simulink model "W06_city_highway_cs"  (R2019a)
settings: Solver=ode5  StartTime=0.0  StopTime=inf  FixedStep=1/60  RelTol=1e-3
PreLoadFcn:
  | mbxruntime.callbacks.PreLoadFcn(bdroot);
PostLoadFcn:
  | mbxruntime.callbacks.PostLoadFcn(bdroot);
InitFcn:
  | mbxruntime.callbacks.InitFcn(bdroot);
StartFcn:
  | mbxruntime.callbacks.StartFcn(bdroot);
StopFcn:
  | mbxruntime.callbacks.StopFcn(bdroot);
model workspace: external: MAT-File .\W06_city_highway_cs_hws.mat (data not in the file)
undefined symbols (not defined in the file or in its folder): DiscIntNeverNeededParam, FovAzimuth, FovAzimuthDefined, FovElevation, FovElevationDefined, Header, InitImageOutputDir, LocationX, LocationXDefined, LocationY, LocationYDefined, LocationZ, LocationZDefined, Orientation, OrientationPitch, OrientationPitchDefined, OrientationRoll, OrientationRollDefined, OrientationYaw, OrientationYawDefined, Poses, Poses_SL_Info, Position, W06_city_highway_cs_0270c22595f3b0e3, W06_city_highway_cs_086892688dd32ddc, W06_city_highway_cs_328c49ac39fca66b, W06_city_highway_cs_35ce05381b8ebe8c, W06_city_highway_cs_47b384f162638175, W06_city_highway_cs_766f76ce4de94dd5, W06_city_highway_cs_8c547f67cb81ffba, W06_city_highway_cs_aed52f2a7724a4f9, W06_city_highway_cs_Audi_A8_Sedan_1_Path_pathUniqueID, W06_city_highway_cs_b74cbb1f9f7331b5, W06_city_highway_cs_Citroen_C3_Hatchback_1_Path_pathUniqueID, W06_city_highway_cs_d395f8835e0c28b3, W06_city_highway_cs_e5f9d1759e19e2b4, W06_city_highway_cs_Toyota_Previa_MPV_1_Path_pathUniqueID
libraries: adeye_lib x26, simulink_extras x24, robotlib x7, sharedtransform x4, PreScanSimulinkLibrary x2, PreScanUsefulBlocks x1
(part 8 of 8)

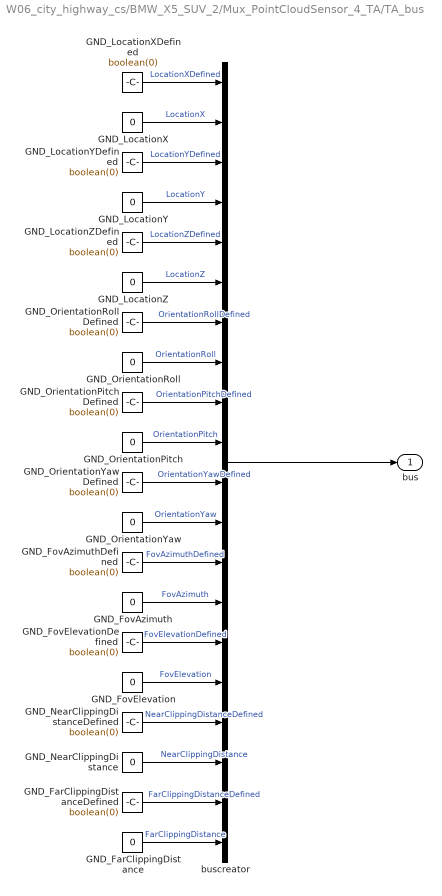
== system W06_city_highway_cs/BMW_X5_SUV_2/Mux_PointCloudSensor_4_TA/TA_bus ==
  GND_FarClippingDistance : Constant  Value=0
  GND_FarClippingDistanceDefined : Constant  Value=boolean(0)
  GND_FovAzimuth : Constant  Value=0
  GND_FovAzimuthDefined : Constant  Value=boolean(0)
  GND_FovElevation : Constant  Value=0
  GND_FovElevationDefined : Constant  Value=boolean(0)
  GND_LocationX : Constant  Value=0
  GND_LocationXDefined : Constant  Value=boolean(0)
  GND_LocationY : Constant  Value=0
  GND_LocationYDefined : Constant  Value=boolean(0)
  GND_LocationZ : Constant  Value=0
  GND_LocationZDefined : Constant  Value=boolean(0)
  GND_NearClippingDistance : Constant  Value=0
  GND_NearClippingDistanceDefined : Constant  Value=boolean(0)
  GND_OrientationPitch : Constant  Value=0
  GND_OrientationPitchDefined : Constant  Value=boolean(0)
  GND_OrientationRoll : Constant  Value=0
  GND_OrientationRollDefined : Constant  Value=boolean(0)
  GND_OrientationYaw : Constant  Value=0
  GND_OrientationYawDefined : Constant  Value=boolean(0)
  buscreator : BusCreator  Inputs=20  OutDataTypeStr=Bus: PRESCAN_PCS_TA_DATA  NonVirtualBus=on
  bus : Outport  OutDataTypeStr=Bus: PRESCAN_PCS_TA_DATA
  wires:
  GND_LocationXDefined/1 -> buscreator/1  "LocationXDefined"
  GND_LocationX/1 -> buscreator/2  "LocationX"
  GND_LocationYDefined/1 -> buscreator/3  "LocationYDefined"
  GND_LocationY/1 -> buscreator/4  "LocationY"
  GND_LocationZDefined/1 -> buscreator/5  "LocationZDefined"
  GND_LocationZ/1 -> buscreator/6  "LocationZ"
  GND_OrientationRollDefined/1 -> buscreator/7  "OrientationRollDefined"
  GND_OrientationRoll/1 -> buscreator/8  "OrientationRoll"
  GND_OrientationPitchDefined/1 -> buscreator/9  "OrientationPitchDefined"
  GND_OrientationPitch/1 -> buscreator/10  "OrientationPitch"
  GND_OrientationYawDefined/1 -> buscreator/11  "OrientationYawDefined"
  GND_OrientationYaw/1 -> buscreator/12  "OrientationYaw"
  GND_FovAzimuthDefined/1 -> buscreator/13  "FovAzimuthDefined"
  GND_FovAzimuth/1 -> buscreator/14  "FovAzimuth"
  GND_FovElevationDefined/1 -> buscreator/15  "FovElevationDefined"
  GND_FovElevation/1 -> buscreator/16  "FovElevation"
  GND_NearClippingDistanceDefined/1 -> buscreator/17  "NearClippingDistanceDefined"
  GND_NearClippingDistance/1 -> buscreator/18  "NearClippingDistance"
  GND_FarClippingDistanceDefined/1 -> buscreator/19  "FarClippingDistanceDefined"
  GND_FarClippingDistance/1 -> buscreator/20  "FarClippingDistance"
  buscreator/1 -> bus/1

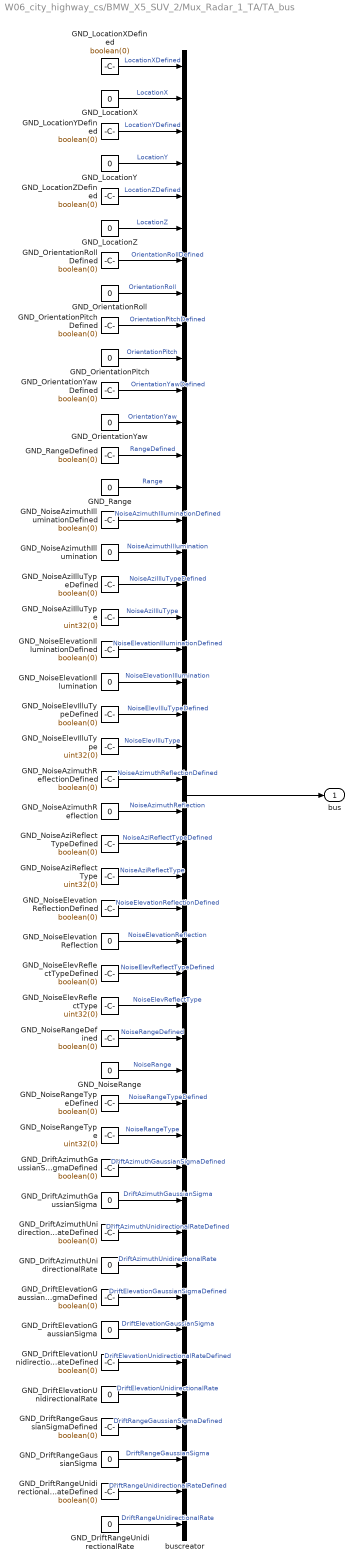
== system W06_city_highway_cs/BMW_X5_SUV_2/Mux_Radar_1_TA/TA_bus ==
  GND_DriftAzimuthGaussianSigma : Constant  Value=0
  GND_DriftAzimuthGaussianSigmaDefined : Constant  Value=boolean(0)
  GND_DriftAzimuthUnidirectionalRate : Constant  Value=0
  GND_DriftAzimuthUnidirectionalRateDefined : Constant  Value=boolean(0)
  GND_DriftElevationGaussianSigma : Constant  Value=0
  GND_DriftElevationGaussianSigmaDefined : Constant  Value=boolean(0)
  GND_DriftElevationUnidirectionalRate : Constant  Value=0
  GND_DriftElevationUnidirectionalRateDefined : Constant  Value=boolean(0)
  GND_DriftRangeGaussianSigma : Constant  Value=0
  GND_DriftRangeGaussianSigmaDefined : Constant  Value=boolean(0)
  GND_DriftRangeUnidirectionalRate : Constant  Value=0
  GND_DriftRangeUnidirectionalRateDefined : Constant  Value=boolean(0)
  GND_LocationX : Constant  Value=0
  GND_LocationXDefined : Constant  Value=boolean(0)
  GND_LocationY : Constant  Value=0
  GND_LocationYDefined : Constant  Value=boolean(0)
  GND_LocationZ : Constant  Value=0
  GND_LocationZDefined : Constant  Value=boolean(0)
  GND_NoiseAziIlluType : Constant  Value=uint32(0)
  GND_NoiseAziIlluTypeDefined : Constant  Value=boolean(0)
  GND_NoiseAziReflectType : Constant  Value=uint32(0)
  GND_NoiseAziReflectTypeDefined : Constant  Value=boolean(0)
  GND_NoiseAzimuthIllumination : Constant  Value=0
  GND_NoiseAzimuthIlluminationDefined : Constant  Value=boolean(0)
  GND_NoiseAzimuthReflection : Constant  Value=0
  GND_NoiseAzimuthReflectionDefined : Constant  Value=boolean(0)
  GND_NoiseElevIlluType : Constant  Value=uint32(0)
  GND_NoiseElevIlluTypeDefined : Constant  Value=boolean(0)
  GND_NoiseElevReflectType : Constant  Value=uint32(0)
  GND_NoiseElevReflectTypeDefined : Constant  Value=boolean(0)
  GND_NoiseElevationIllumination : Constant  Value=0
  GND_NoiseElevationIlluminationDefined : Constant  Value=boolean(0)
  GND_NoiseElevationReflection : Constant  Value=0
  GND_NoiseElevationReflectionDefined : Constant  Value=boolean(0)
  GND_NoiseRange : Constant  Value=0
  GND_NoiseRangeDefined : Constant  Value=boolean(0)
  GND_NoiseRangeType : Constant  Value=uint32(0)
  GND_NoiseRangeTypeDefined : Constant  Value=boolean(0)
  GND_OrientationPitch : Constant  Value=0
  GND_OrientationPitchDefined : Constant  Value=boolean(0)
  GND_OrientationRoll : Constant  Value=0
  GND_OrientationRollDefined : Constant  Value=boolean(0)
  GND_OrientationYaw : Constant  Value=0
  GND_OrientationYawDefined : Constant  Value=boolean(0)
  GND_Range : Constant  Value=0
  GND_RangeDefined : Constant  Value=boolean(0)
  buscreator : BusCreator  Inputs=46  OutDataTypeStr=Bus: PRESCAN_SCANNERSENSOR_TA  NonVirtualBus=on
  bus : Outport  OutDataTypeStr=Bus: PRESCAN_SCANNERSENSOR_TA
  wires:
  GND_LocationXDefined/1 -> buscreator/1  "LocationXDefined"
  GND_LocationX/1 -> buscreator/2  "LocationX"
  GND_LocationYDefined/1 -> buscreator/3  "LocationYDefined"
  GND_LocationY/1 -> buscreator/4  "LocationY"
  GND_LocationZDefined/1 -> buscreator/5  "LocationZDefined"
  GND_LocationZ/1 -> buscreator/6  "LocationZ"
  GND_OrientationRollDefined/1 -> buscreator/7  "OrientationRollDefined"
  GND_OrientationRoll/1 -> buscreator/8  "OrientationRoll"
  GND_OrientationPitchDefined/1 -> buscreator/9  "OrientationPitchDefined"
  GND_OrientationPitch/1 -> buscreator/10  "OrientationPitch"
  GND_OrientationYawDefined/1 -> buscreator/11  "OrientationYawDefined"
  GND_OrientationYaw/1 -> buscreator/12  "OrientationYaw"
  GND_RangeDefined/1 -> buscreator/13  "RangeDefined"
  GND_Range/1 -> buscreator/14  "Range"
  GND_NoiseAzimuthIlluminationDefined/1 -> buscreator/15  "NoiseAzimuthIlluminationDefined"
  GND_NoiseAzimuthIllumination/1 -> buscreator/16  "NoiseAzimuthIllumination"
  GND_NoiseAziIlluTypeDefined/1 -> buscreator/17  "NoiseAziIlluTypeDefined"
  GND_NoiseAziIlluType/1 -> buscreator/18  "NoiseAziIlluType"
  GND_NoiseElevationIlluminationDefined/1 -> buscreator/19  "NoiseElevationIlluminationDefined"
  GND_NoiseElevationIllumination/1 -> buscreator/20  "NoiseElevationIllumination"
  GND_NoiseElevIlluTypeDefined/1 -> buscreator/21  "NoiseElevIlluTypeDefined"
  GND_NoiseElevIlluType/1 -> buscreator/22  "NoiseElevIlluType"
  GND_NoiseAzimuthReflectionDefined/1 -> buscreator/23  "NoiseAzimuthReflectionDefined"
  GND_NoiseAzimuthReflection/1 -> buscreator/24  "NoiseAzimuthReflection"
  GND_NoiseAziReflectTypeDefined/1 -> buscreator/25  "NoiseAziReflectTypeDefined"
  GND_NoiseAziReflectType/1 -> buscreator/26  "NoiseAziReflectType"
  GND_NoiseElevationReflectionDefined/1 -> buscreator/27  "NoiseElevationReflectionDefined"
  GND_NoiseElevationReflection/1 -> buscreator/28  "NoiseElevationReflection"
  GND_NoiseElevReflectTypeDefined/1 -> buscreator/29  "NoiseElevReflectTypeDefined"
  GND_NoiseElevReflectType/1 -> buscreator/30  "NoiseElevReflectType"
  GND_NoiseRangeDefined/1 -> buscreator/31  "NoiseRangeDefined"
  GND_NoiseRange/1 -> buscreator/32  "NoiseRange"
  GND_NoiseRangeTypeDefined/1 -> buscreator/33  "NoiseRangeTypeDefined"
  GND_NoiseRangeType/1 -> buscreator/34  "NoiseRangeType"
  GND_DriftAzimuthGaussianSigmaDefined/1 -> buscreator/35  "DriftAzimuthGaussianSigmaDefined"
  GND_DriftAzimuthGaussianSigma/1 -> buscreator/36  "DriftAzimuthGaussianSigma"
  GND_DriftAzimuthUnidirectionalRateDefined/1 -> buscreator/37  "DriftAzimuthUnidirectionalRateDefined"
  GND_DriftAzimuthUnidirectionalRate/1 -> buscreator/38  "DriftAzimuthUnidirectionalRate"
  GND_DriftElevationGaussianSigmaDefined/1 -> buscreator/39  "DriftElevationGaussianSigmaDefined"
  GND_DriftElevationGaussianSigma/1 -> buscreator/40  "DriftElevationGaussianSigma"
  GND_DriftElevationUnidirectionalRateDefined/1 -> buscreator/41  "DriftElevationUnidirectionalRateDefined"
  GND_DriftElevationUnidirectionalRate/1 -> buscreator/42  "DriftElevationUnidirectionalRate"
  GND_DriftRangeGaussianSigmaDefined/1 -> buscreator/43  "DriftRangeGaussianSigmaDefined"
  GND_DriftRangeGaussianSigma/1 -> buscreator/44  "DriftRangeGaussianSigma"
  GND_DriftRangeUnidirectionalRateDefined/1 -> buscreator/45  "DriftRangeUnidirectionalRateDefined"
  GND_DriftRangeUnidirectionalRate/1 -> buscreator/46  "DriftRangeUnidirectionalRate"
  buscreator/1 -> bus/1

== system W06_city_highway_cs/BMW_X5_SUV_2/SELF_Demux/compas converter ==
  rotz [rad] : Inport
  cart2compas : Subsystem
  rad2deg : Gain  Gain=180/pi
  heading [deg] : Outport
  wires:
  rad2deg/1 -> cart2compas/1(Angle [deg])
  rotz [rad]/1 -> rad2deg/1
  cart2compas/1(heading [deg]) -> heading [deg]/1

== system W06_city_highway_cs/Citroen_C3_Hatchback_1/SELF_Demux/compas converter ==
  rotz [rad] : Inport
  cart2compas : Subsystem
  rad2deg : Gain  Gain=180/pi
  heading [deg] : Outport
  wires:
  rad2deg/1 -> cart2compas/1(Angle [deg])
  rotz [rad]/1 -> rad2deg/1
  cart2compas/1(heading [deg]) -> heading [deg]/1

== system W06_city_highway_cs/MercedesBenz_Actros_2541_L_6x2_1/SELF_Demux/compas converter ==
  rotz [rad] : Inport
  cart2compas : Subsystem
  rad2deg : Gain  Gain=180/pi
  heading [deg] : Outport
  wires:
  rad2deg/1 -> cart2compas/1(Angle [deg])
  rotz [rad]/1 -> rad2deg/1
  cart2compas/1(heading [deg]) -> heading [deg]/1

== system W06_city_highway_cs/Toyota_Previa_MPV_1/SELF_Demux/compas converter ==
  rotz [rad] : Inport
  cart2compas : Subsystem
  rad2deg : Gain  Gain=180/pi
  heading [deg] : Outport
  wires:
  rad2deg/1 -> cart2compas/1(Angle [deg])
  rotz [rad]/1 -> rad2deg/1
  cart2compas/1(heading [deg]) -> heading [deg]/1

== system W06_city_highway_cs/Audi_A8_Sedan_1/SELF_Demux/compas converter/cart2compas ==
  Angle [deg] : Inport
  Constant : Constant  Value=90
  Constant1 : Constant  Value=360
  Gain : Gain  Gain=1/360
  Gain1 : Gain  Gain=360
  Gain2 : Gain  Gain=-1
  Rounding Function : Rounding
  Sum : Sum  Inputs=|-+
  Sum1 : Sum  Inputs=-+|
  Sum2 : Sum  Inputs=++|
  heading [deg] : Outport
  wires:
  Gain/1 -> Rounding Function/1
  Rounding Function/1 -> Gain1/1
  Gain1/1 -> Sum/1
  Angle [deg]/1 -> Sum1/2
  Sum/1 -> Gain2/1
  Sum1/1 -> Gain/1, Sum/2
  Constant/1 -> Sum1/1
  Gain2/1 -> Sum2/2
  Constant1/1 -> Sum2/1
  Sum2/1 -> heading [deg]/1

== system W06_city_highway_cs/BMW_X5_SUV_2/Dynamics_Empty/Subsystem/If Action Subsystem ==
  In1 : Inport
  In2 : Inport  Port=2
  Action Port : ActionPort  ActionPortLabel=if(u1 > u2)
  Add : Sum
  Out1 : Outport
  wires:
  Add/1 -> Out1/1
  In1/1 -> Add/1
  In2/1 -> Add/2

== system W06_city_highway_cs/BMW_X5_SUV_2/Dynamics_Empty/Subsystem/If Action Subsystem1 ==
  In1 : Inport
  In2 : Inport  Port=2
  Action Port : ActionPort  ActionPortLabel=else
  Add : Sum  Inputs=+-
  Out1 : Outport
  wires:
  Add/1 -> Out1/1
  In2/1 -> Add/2
  In1/1 -> Add/1

== system W06_city_highway_cs/BMW_X5_SUV_2/Dynamics_Empty/Subsystem/If Action Subsystem2 ==
  In1 : Inport
  Action Port : ActionPort  ActionPortLabel=elseif(u1 > -u2)
  Out1 : Outport
  wires:
  In1/1 -> Out1/1

== system W06_city_highway_cs/BMW_X5_SUV_2/SELF_Demux/compas converter/cart2compas ==
  Angle [deg] : Inport
  Constant : Constant  Value=90
  Constant1 : Constant  Value=360
  Gain : Gain  Gain=1/360
  Gain1 : Gain  Gain=360
  Gain2 : Gain  Gain=-1
  Rounding Function : Rounding
  Sum : Sum  Inputs=|-+
  Sum1 : Sum  Inputs=-+|
  Sum2 : Sum  Inputs=++|
  heading [deg] : Outport
  wires:
  Gain/1 -> Rounding Function/1
  Rounding Function/1 -> Gain1/1
  Gain1/1 -> Sum/1
  Angle [deg]/1 -> Sum1/2
  Sum/1 -> Gain2/1
  Sum1/1 -> Gain/1, Sum/2
  Constant/1 -> Sum1/1
  Gain2/1 -> Sum2/2
  Constant1/1 -> Sum2/1
  Sum2/1 -> heading [deg]/1

== system W06_city_highway_cs/Citroen_C3_Hatchback_1/SELF_Demux/compas converter/cart2compas ==
  Angle [deg] : Inport
  Constant : Constant  Value=90
  Constant1 : Constant  Value=360
  Gain : Gain  Gain=1/360
  Gain1 : Gain  Gain=360
  Gain2 : Gain  Gain=-1
  Rounding Function : Rounding
  Sum : Sum  Inputs=|-+
  Sum1 : Sum  Inputs=-+|
  Sum2 : Sum  Inputs=++|
  heading [deg] : Outport
  wires:
  Gain/1 -> Rounding Function/1
  Rounding Function/1 -> Gain1/1
  Gain1/1 -> Sum/1
  Angle [deg]/1 -> Sum1/2
  Sum/1 -> Gain2/1
  Sum1/1 -> Gain/1, Sum/2
  Constant/1 -> Sum1/1
  Gain2/1 -> Sum2/2
  Constant1/1 -> Sum2/1
  Sum2/1 -> heading [deg]/1

== system W06_city_highway_cs/MercedesBenz_Actros_2541_L_6x2_1/SELF_Demux/compas converter/cart2compas ==
  Angle [deg] : Inport
  Constant : Constant  Value=90
  Constant1 : Constant  Value=360
  Gain : Gain  Gain=1/360
  Gain1 : Gain  Gain=360
  Gain2 : Gain  Gain=-1
  Rounding Function : Rounding
  Sum : Sum  Inputs=|-+
  Sum1 : Sum  Inputs=-+|
  Sum2 : Sum  Inputs=++|
  heading [deg] : Outport
  wires:
  Gain/1 -> Rounding Function/1
  Rounding Function/1 -> Gain1/1
  Gain1/1 -> Sum/1
  Angle [deg]/1 -> Sum1/2
  Sum/1 -> Gain2/1
  Sum1/1 -> Gain/1, Sum/2
  Constant/1 -> Sum1/1
  Gain2/1 -> Sum2/2
  Constant1/1 -> Sum2/1
  Sum2/1 -> heading [deg]/1

== system W06_city_highway_cs/Toyota_Previa_MPV_1/SELF_Demux/compas converter/cart2compas ==
  Angle [deg] : Inport
  Constant : Constant  Value=90
  Constant1 : Constant  Value=360
  Gain : Gain  Gain=1/360
  Gain1 : Gain  Gain=360
  Gain2 : Gain  Gain=-1
  Rounding Function : Rounding
  Sum : Sum  Inputs=|-+
  Sum1 : Sum  Inputs=-+|
  Sum2 : Sum  Inputs=++|
  heading [deg] : Outport
  wires:
  Gain/1 -> Rounding Function/1
  Rounding Function/1 -> Gain1/1
  Gain1/1 -> Sum/1
  Angle [deg]/1 -> Sum1/2
  Sum/1 -> Gain2/1
  Sum1/1 -> Gain/1, Sum/2
  Constant/1 -> Sum1/1
  Gain2/1 -> Sum2/2
  Constant1/1 -> Sum2/1
  Sum2/1 -> heading [deg]/1
